simulink model "test_sample"  (R2022b)
settings: Solver=ode4  StartTime=0.0  StopTime=10.0  FixedStep=0.001  RelTol=1e-3
values from neighbouring files (symbols this model uses):
  k = -3    [untitled2.m]
  k1 = 4    [untitled2.m]
settings Model: Creator=user  LastModifiedBy=user
settings DataIOCC: ReturnWorkspaceOutputs=off

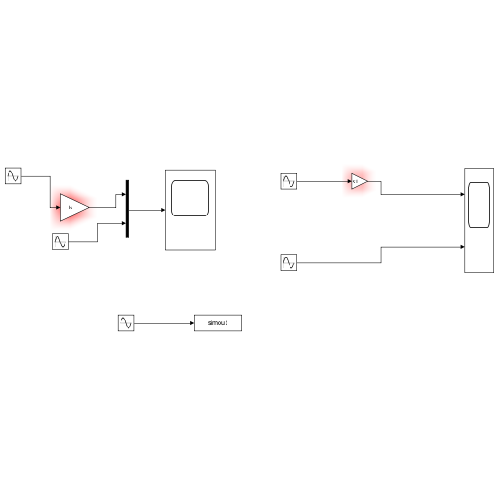
[thumbnail: Simulink's stored preview of the top-level diagram]
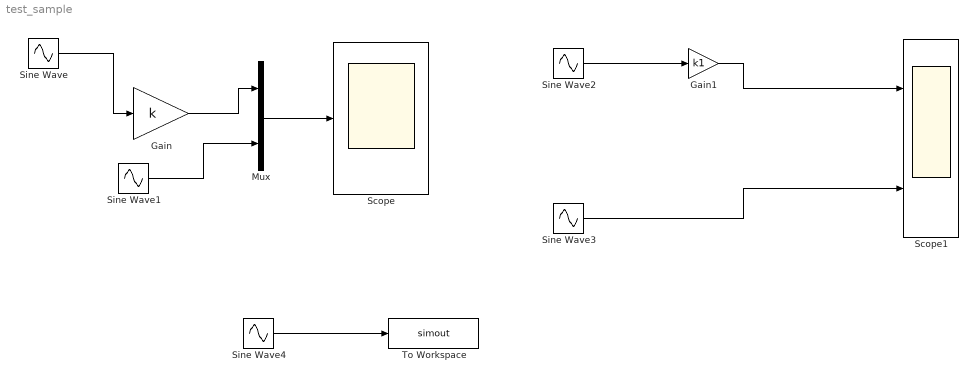
== system test_sample ==
  Gain : Gain  Gain=k
  Gain1 : Gain  Gain=k1
  Mux : Mux  Inputs=2
  Scope : Scope
  Scope1 : Scope  NumInputPorts=2
  Sine Wave : Sin  SampleTime=0
  Sine Wave1 : Sin  Phase=pi/2  SampleTime=0
  Sine Wave2 : Sin  SampleTime=0
  Sine Wave3 : Sin  Phase=pi/2  SampleTime=0
  Sine Wave4 : Sin  Phase=pi/2  SampleTime=0
  To Workspace : ToWorkspace  VariableName=simout  SaveFormat=Timeseries  SampleTime=-1
  wires:
  Mux/1 -> Scope/1
  Sine Wave/1 -> Gain/1
  Sine Wave1/1 -> Mux/2
  Sine Wave3/1 -> Scope1/2
  Sine Wave4/1 -> To Workspace/1
  Gain/1 -> Mux/1
  Sine Wave2/1 -> Gain1/1
  Gain1/1 -> Scope1/1
